simulink model "single_phase_bridge_controlled_rectifier"  (R2023b)
settings: Solver=VariableStepAuto  StartTime=0.0  StopTime=0.1  MaxStep=1e-4  RelTol=1e-3
libraries: spsThyristorLib x4, spsSeriesRLCBranchLib x1, spsMultimeterLib x1, spsACVoltageSourceLib x1, sps_lib x1
settings Model: Creator=LuvB4  LastModifiedBy=LuvB4

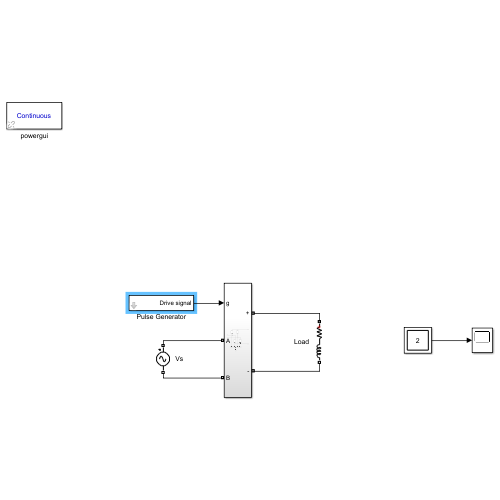
[thumbnail: Simulink's stored preview of the top-level diagram]
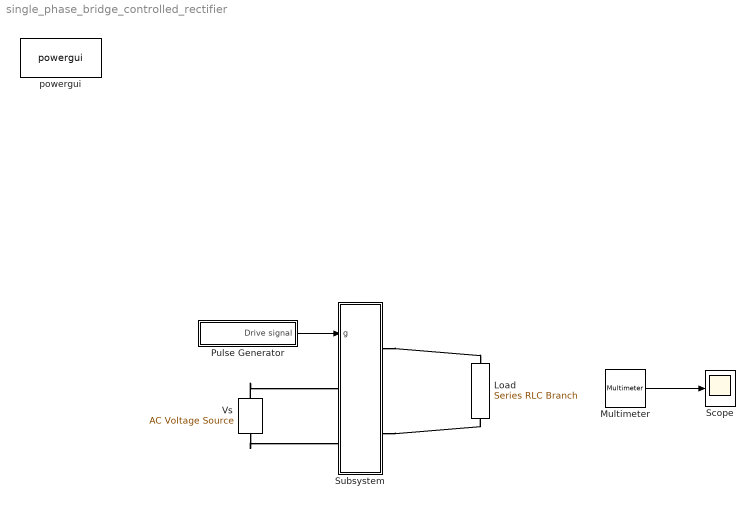
== system single_phase_bridge_controlled_rectifier ==
  Load : spsSeriesRLCBranchLib/Series RLC Branch  LConnTagsString=__new0  RConnTagsString=__new0  BranchType=RL  Resistance=10  Inductance=10/(2*pi*50)  SetiL0=off  InitialCurrent=0  Capacitance=1e-6  Setx0=off  InitialVoltage=0  Measurements=Branch voltage and current
  Multimeter : spsMultimeterLib/Multimeter  L=3  sel=[1 3]  yselected={}  Gain=[1 1]  OutputType=Complex  PlotAtSimulationStop=off  PhasorSimulation=off
  Pulse Generator : Subsystem  mask{freq=50, alpha=45}
      mask prompts: freq "Grid frequent"
      mask DialogControl DescGroupVar Prompt: %<MaskType>Pulse Generator
      mask DialogControl DescTextVar Prompt: %<MaskDescription>Simple pulse generator mask test
      mask DialogControl ParameterGroupVar Prompt: 参数
  Scope : Scope
  Subsystem : Subsystem
  Vs : spsACVoltageSourceLib/AC Voltage Source  Amplitude=220*sqrt(2)  Phase=0  Frequency=50  SampleTime=0  Measurements=Voltage  BusType=swing  Pref=10e3  Qref=0  Qmin=-inf  Qmax=+inf
  powergui : sps_lib/powergui  Priority=1  SimulationMode=Continuous  SampleTime=50e-6  frequency=60  Iterations=50  frequencyindice=50  Pbase=100e6  ErrMax=1e-4  UnitsV=kV  UnitsW=MW  buscounter=0  FunctionMessages=off  echomessages=off  EnableUseOfTLC=off  CurrentSourceSwitches=off  DisableSnubberDevices=off  DisableRonSwitches=off  DisableVfSwitches=off  DisplayEquations=off  AutomaticDiscreteSolvers=off  SolverType=Tustin/Backward Euler (TBE)  Interpol=off  ExternalGateDelay=off  methode=off  Ts=100  x0status=blocks  SPID=on  SwTol=0  HookPort=off  NonlinearTolerance=1e-4  nMaxIteration=100  ContinueOnMaxIteration=off  RestoreLinks=warning  ResistiveCurrentMeasurement=off  Frange=[0:2:500]  Ylog=off  Xlog=on  ShowGrid=off  save=off  variable=ZData  structure=0  ZoomFFT=off  StartTime=0.0  cycles=1  DisplayStyle=1  fundamental=60  FreqAxis=off  MaxFrequency=1000  frequencyindicesteady=1  RmsSteady=1  display=off
  wires:
  Pulse Generator/1(Drive signal) -> Subsystem/1(g)
  Multimeter/1 -> Scope/1
  connections:
  Subsystem/RConn1 -- Load/LConn1
  Subsystem/RConn2 -- Load/RConn1
  Vs/RConn1 -- Subsystem/LConn1
  Vs/LConn1 -- Subsystem/LConn2

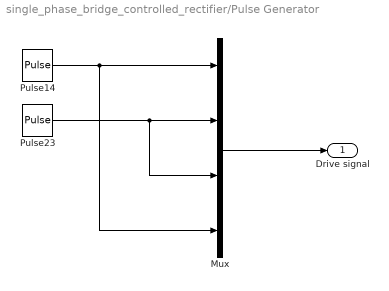
== system single_phase_bridge_controlled_rectifier/Pulse Generator ==
  Mux : Mux
  Pulse14 : DiscretePulseGenerator  PulseType=Time based  Period=1/freq  PulseWidth=5  PhaseDelay=(alpha/360)*(1/freq)
  Pulse23 : DiscretePulseGenerator  PulseType=Time based  Period=1/freq  PulseWidth=5  PhaseDelay=((alpha+180)/360)*(1/freq)
  Drive signal : Outport
  wires:
  Mux/1 -> Drive signal/1
  Pulse14/1 -> Mux/4, Mux/1
  Pulse23/1 -> Mux/3, Mux/2

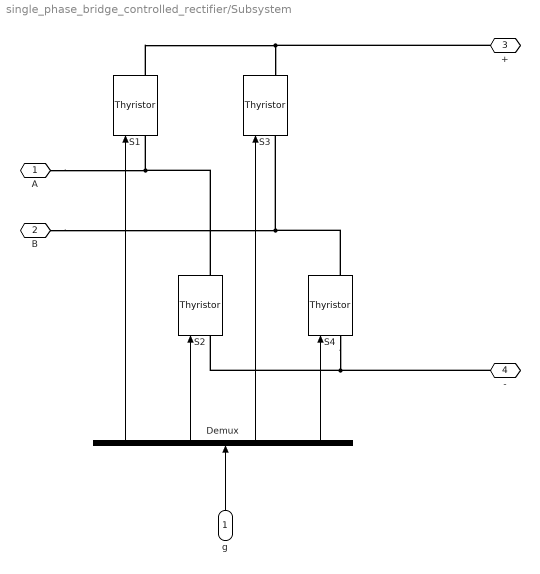
== system single_phase_bridge_controlled_rectifier/Subsystem ==
  g : Inport
  Demux : Demux
  S{1..4} (4 alike) : spsThyristorLib/Thyristor  Ron=0.001  Lon=0  Vf=0  IC=0  Rs=0  Cs=0  Measurements=on
  A : PMIOPort  Side=Left
  B : PMIOPort  Port=2  Side=Left
  + : PMIOPort  Port=3  Side=Right
  - : PMIOPort  Port=4  Side=Right
  wires:
  g/1 -> Demux/1
  Demux/1 -> S1/1
  Demux/2 -> S2/1
  Demux/3 -> S3/1
  Demux/4 -> S4/1
  connections:
  S1/RConn1 -- +/RConn1 -- S3/RConn1
  S2/RConn1 -- A/RConn1 -- S1/LConn1
  S4/LConn1 -- -/RConn1 -- S2/LConn1
  S4/RConn1 -- B/RConn1 -- S3/LConn1
